simulink model "validation1"  (R2025a)
settings: Solver=VariableStepAuto  StartTime=0.0  StopTime=10.0  RelTol=1e-3
settings Model: Creator=Admin  LastModifiedBy=Admin

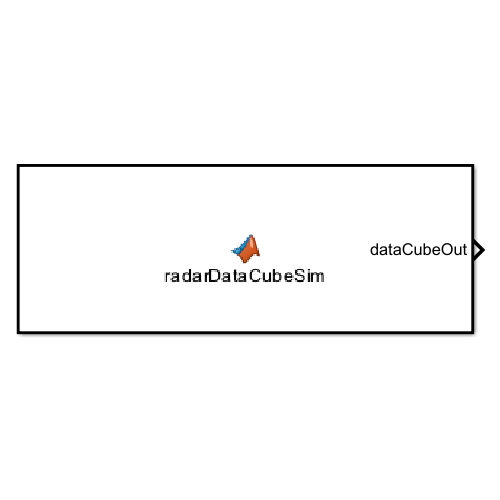
[thumbnail: Simulink's stored preview of the top-level diagram]
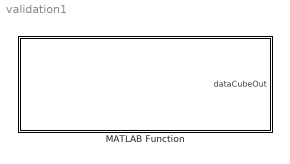
== system validation1 ==
  MATLAB Function : MATLAB Function  TreatAsAtomicUnit=on

== matlab function validation1/MATLAB Function ==
  data: dataCubeOut output
function dataCubeOut = radarDataCubeSim()
%#codegen
% Simulink-compatible function to generate radar data cube with matched filtering

%% === Parameters ===
numPulses   = 64;       % Number of pulses (slow time)
numChannels = 8;        % Number of array elements
fc          = 1e9;      % Carrier frequency (Hz)
c           = physconst('LightSpeed');
fs          = 20e6;     % Sampling frequency
PRF         = 10e3;     % Pulse Repetition Frequency
pw          = 33e-6;    % Pulse width
tx_gain     = 20;       % dB
peakPower   = 5000;     % W
target_range= 10000;    % m
target_rcs  = 5;        % m²

%% === Array & Waveform ===
antenna = phased.IsotropicAntennaElement( ...
    'FrequencyRange',[800e6 1.2e9]);
array = phased.ULA('NumElements',numChannels, ...
    'ElementSpacing',0.5*(c/fc),'Element',antenna);

waveform = phased.RectangularWaveform( ...
    'SampleRate',fs,'PRF',PRF,'PulseWidth',pw);

%% === Radar Components ===
transmitter = phased.Transmitter( ...
    'Gain',tx_gain,'PeakPower',peakPower);

target = phased.RadarTarget( ...
    'MeanRCS',target_rcs,'OperatingFrequency',fc);

channel = phased.FreeSpace( ...
    'SampleRate',fs,'TwoWayPropagation',false, ...
    'OperatingFrequency',fc);

collector = phased.Collector('Sensor',array, ...
    'OperatingFrequency',fc);

receiver = phased.ReceiverPreamp( ...
    'Gain',0,'NoiseFigure',0,'SampleRate',fs);

%% === Matched Filter (for pulse compression) ===
mf = phased.MatchedFilter('Coefficients',getMatchedFilter(waveform));

%% === Data Cube Initialization ===
samplesPerPulse = round(fs/PRF);
dataCube = complex(zeros(samplesPerPulse,numPulses,numChannels));

%% === Positions and Velocities ===
radarPos   = [0;0;0];
radarVel   = [0;0;0];
targetPos  = [target_range;0;0];
targetVel  = [0;0;0];

%% === Loop over pulses ===
for p = 1:numPulses
    % Generate one pulse
    sig = waveform();
    txsig = transmitter(sig);

    % Propagate to target
    propSig = channel(txsig,radarPos,targetPos,radarVel,targetVel);

    % Reflection
    reflSig = target(propSig);

    % Back to radar
    rxSig = channel(reflSig,targetPos,radarPos,targetVel,radarVel);

    % Array collection
    collected = collector(rxSig,[0;0]);

    % Receiver front-end
    rx = receiver(collected);

    % Matched filtering
    mfOut = mf(rx);

    % Store into cube
    dataCube(:,p,:) = mfOut(1:samplesPerPulse,:);
end

%% === Output ===
dataCubeOut = dataCube;

end
